simulink model "bolustry"  (R2023b)
settings: Solver=VariableStepAuto  StartTime=0.0  StopTime=10.0  RelTol=1e-3
settings Model: Creator=anson  LastModifiedBy=anson

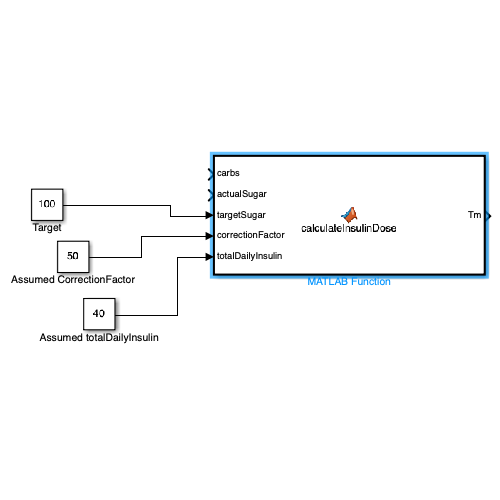
[thumbnail: Simulink's stored preview of the top-level diagram]
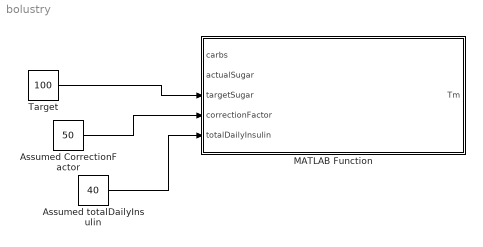
== system bolustry ==
  Assumed CorrectionFactor : Constant  Value=50
  Assumed totalDailyInsulin : Constant  Value=40
  MATLAB Function : MATLAB Function  TreatAsAtomicUnit=on
  Target : Constant  Value=100
  wires:
  Assumed CorrectionFactor/1 -> MATLAB Function/4(correctionFactor)
  Target/1 -> MATLAB Function/3(targetSugar)
  Assumed totalDailyInsulin/1 -> MATLAB Function/5(totalDailyInsulin)

== matlab function bolustry/MATLAB Function ==
  data: carbs input; Tm output; actualSugar input; targetSugar input; correctionFactor input; totalDailyInsulin input
function Tm = calculateInsulinDose(carbs, actualSugar, targetSugar, correctionFactor, totalDailyInsulin)
    % Carbohydrate meal coverage
    insulinToCarbRatio = 500 / totalDailyInsulin; % Rule of 500
    CMC = carbs / insulinToCarbRatio; % Carbohydrate coverage dose

    % High Blood Sugar Correction
    deltaSugar = actualSugar - targetSugar;
    CD = deltaSugar / correctionFactor; % Correction dose for high blood sugar

    % Total meal insulin dose
    Tm = CMC + CD; % Total meal insulin dose
end
